simulink model "Hierarchical_Scheduler_OpenLoop"  (Simulink 7.3)
settings: Solver=ode45  StartTime=0.0  StopTime=30.0  RelTol=1e-3
undefined symbols (not defined in the file or in its folder): DiscIntNeverNeededParam
settings Model: Creator=nmd01  LastModifiedBy=nmd01

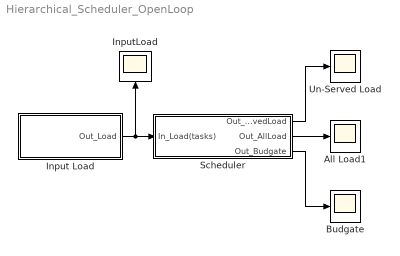
== system Hierarchical_Scheduler_OpenLoop ==
  All Load1 : Scope
      settings: SaveName=Utilization1  DataFormat=Array
  Budgate : Scope
      settings: SaveName=Utilization2  DataFormat=Array
  Input Load : Subsystem
  InputLoad : Scope
      settings: SaveName=Utilization3  DataFormat=Array
  Scheduler : Subsystem
  Un-Served Load : Scope
      settings: SaveName=Utilization  DataFormat=Array
  wires:
  Input Load/1(Out_Load) -> Scheduler/1(In_Load(tasks)), InputLoad/1
  Scheduler/1(Out_Un-servedLoad) -> Un-Served Load/1
  Scheduler/2(Out_AllLoad) -> All Load1/1
  Scheduler/3(Out_Budgate) -> Budgate/1

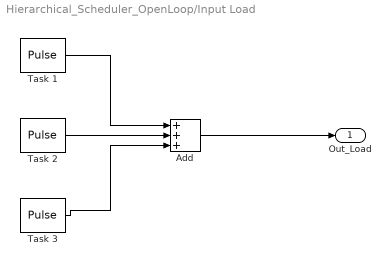
== system Hierarchical_Scheduler_OpenLoop/Input Load ==
  Add : Sum  Inputs=+++  OutDataType=fixdt(1, 16)  OutScaling=2^-10
  Task 1 : DiscretePulseGenerator  PulseType=Time based  Amplitude=3  Period=5  PulseWidth=1  PhaseDelay=0  SampleTime=1
  Task 2 : DiscretePulseGenerator  PulseType=Time based  Amplitude=2  Period=10  PulseWidth=1  PhaseDelay=0  SampleTime=1
  Task 3 : DiscretePulseGenerator  PulseType=Time based  Amplitude=1  Period=8  PulseWidth=1  PhaseDelay=0  SampleTime=1
  Out_Load : Outport  OutDataType=fixdt(1, 16)  OutScaling=2^0
  wires:
  Add/1 -> Out_Load/1
  Task 1/1 -> Add/1
  Task 2/1 -> Add/2
  Task 3/1 -> Add/3

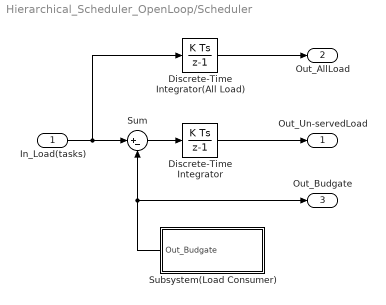
== system Hierarchical_Scheduler_OpenLoop/Scheduler ==
  In_Load(tasks) : Inport  OutDataType=fixdt(1, 16)  OutScaling=2^0
  Discrete-Time Integrator : DiscreteIntegrator  OutDataType=fixdt(1, 16)  OutScaling=2^0  LimitOutput=on  LowerSaturationLimit=0  ICPrevOutput=DiscIntNeverNeededParam  ICPrevScaledInput=DiscIntNeverNeededParam
  Discrete-Time Integrator(All Load) : DiscreteIntegrator  OutDataType=fixdt(1, 16)  OutScaling=2^0  LimitOutput=on  LowerSaturationLimit=0  ICPrevOutput=DiscIntNeverNeededParam  ICPrevScaledInput=DiscIntNeverNeededParam
  Subsystem(Load Consumer) : Subsystem
  Sum : Sum  Inputs=|+-  OutDataType=fixdt(1, 16)  OutScaling=2^0  SampleTime=1
  Out_Un-servedLoad : Outport  OutDataType=fixdt(1, 16)  OutScaling=2^0
  Out_AllLoad : Outport  Port=2  OutDataType=fixdt(1, 16)  OutScaling=2^0
  Out_Budgate : Outport  Port=3  OutDataType=fixdt(1, 16)  OutScaling=2^0
  wires:
  In_Load(tasks)/1 -> Sum/1, Discrete-Time Integrator(All Load)/1
  Sum/1 -> Discrete-Time Integrator/1
  Discrete-Time Integrator/1 -> Out_Un-servedLoad/1
  Subsystem(Load Consumer)/1(Out_Budgate) -> Sum/2, Out_Budgate/1
  Discrete-Time Integrator(All Load)/1 -> Out_AllLoad/1

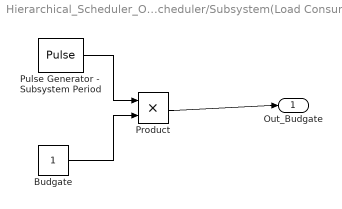
== system Hierarchical_Scheduler_OpenLoop/Scheduler/Subsystem(Load Consumer) ==
  Budgate : Constant  OutDataType=fixdt(1, 16)  OutScaling=2^0
  Product : Product  OutDataType=fixdt(1, 16)  OutScaling=2^0  SampleTime=1  RndMeth=Zero
  Pulse Generator -  Subsystem Period : DiscretePulseGenerator  PulseType=Time based  Amplitude=1  Period=2  PulseWidth=1  PhaseDelay=0  SampleTime=1
  Out_Budgate : Outport  OutDataType=fixdt(1, 16)  OutScaling=2^0
  wires:
  Pulse Generator -  Subsystem Period/1 -> Product/1
  Budgate/1 -> Product/2
  Product/1 -> Out_Budgate/1
